simulink model "enviro"  (R2019b)
settings: Solver=VariableStepAuto  StartTime=0.0  StopTime=10.0  RelTol=1e-3
libraries: aerolibconvert2 x1
settings Model: Creator=Blanca Boado  LastModifiedBy=Blanca Boado

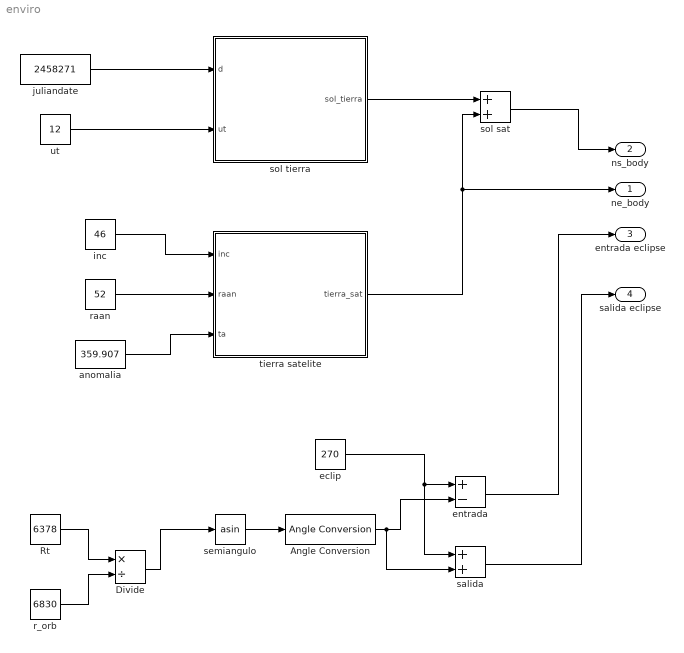
== system enviro ==
  Angle Conversion : aerolibconvert2/Angle Conversion  IU=rad  OU=deg
  Divide : Product  Inputs=*/
  Rt : Constant  Value=6378
  anomalia : Constant  Value=359.907
  eclip : Constant  Value=270
  entrada : Sum  Inputs=+-
  inc : Constant  Value=46
  juliandate : Constant  Value=2458271
  r_orb : Constant  Value=6830
  raan : Constant  Value=52
  salida : Sum
  semiangulo : Trigonometry  Operator=asin
  sol sat : Sum
  sol tierra : MATLAB Function  TreatAsAtomicUnit=on
  tierra satelite : MATLAB Function  TreatAsAtomicUnit=on
  ut : Constant  Value=12
  ne_body : Outport  VectorParamsAs1DForOutWhenUnconnected=off
  ns_body : Outport  Port=2  VectorParamsAs1DForOutWhenUnconnected=off
  entrada eclipse : Outport  Port=3  VectorParamsAs1DForOutWhenUnconnected=off
  salida eclipse : Outport  Port=4  VectorParamsAs1DForOutWhenUnconnected=off
  wires:
  Divide/1 -> semiangulo/1
  entrada/1 -> entrada eclipse/1
  eclip/1 -> salida/1, entrada/1
  salida/1 -> salida eclipse/1
  Rt/1 -> Divide/1
  r_orb/1 -> Divide/2
  sol tierra/1(sol_tierra) -> sol sat/1
  raan/1 -> tierra satelite/2(raan)
  inc/1 -> tierra satelite/1(inc)
  anomalia/1 -> tierra satelite/3(ta)
  semiangulo/1 -> Angle Conversion/1
  Angle Conversion/1 -> salida/2, entrada/2
  tierra satelite/1(tierra_sat) -> ne_body/1, sol sat/2
  sol sat/1 -> ns_body/1
  juliandate/1 -> sol tierra/1(d)
  ut/1 -> sol tierra/2(ut)

== matlab function enviro/tierra satelite ==
  data: tierra_sat output; inc input; raan input; ta input
function tierra_sat = fcn(inc, raan, ta)

R=([cosd(raan) -sind(raan) 0; sind(raan) cosd(raan) 0; 0 0 1]*[1 0 0; 0 cosd(inc) -sind(inc);0 sind(inc) cosd(inc)]);
C_opf=R';
C_opr=[ cosd(ta) sind(ta) 0; -sind(ta) cosd(ta) 0; 0 0 1];
C_lv=[0 1 0;0 0 -1;-1 0 0];
r_lv=[0;0;1];
% r_lv=[0;0;r];
TS=C_opf*C_opr*C_lv*r_lv;


% TS=TS/norm(TS);

tierra_sat=TS;

== matlab function enviro/sol tierra ==
  data: d input; sol_tierra output; ut input
function sol_tierra = fcn(d,ut)

% d=juliandate([2018,month,1,ut,0,0]);
% d=2458271;
T=(d+ut/24-2451545)/36525;

L=mod(280.46+36000.77*T,360);
G=mod(357.528+35999.05*T,360);
lambda=L+1.915*sind(G)+0.02*sind(2*G);
epsilon=23.4393-0.013*T;
E=-1.915*sind(G)-0.02*sind(2*G)+2.4466*sind(2*lambda)-0.053*sind(4*lambda);
GHA=15*ut-180+E;
delta=asind(sind(epsilon)*sind(lambda));
alfa=69; %angulo meridiano punto aries
g2=alfa+GHA;
SD=0.267/(1-0.017*cosd(G));

g1=[cosd(delta) 0 -sind(delta); 0 1 0;sind(delta) 0 cosd(delta)];
g2=[cosd(g2) -sind(g2) 0;sind(g2) cosd(g2) 0; 0 0 1];
v=g1*g2*[1; 0 ;0];

sol_tierra=v;
